simulink model "dspblr7_Ave"  (R2018a)
settings: Solver=VariableStepAuto  StartTime=0.0  StopTime=100e-6  RelTol=1e-3
libraries: xbsIndex_r4 x61, xrbsSSR_Library x17, dspsigattribs x1, hdlsllib x1, simulink x1
(part 2 of 2)

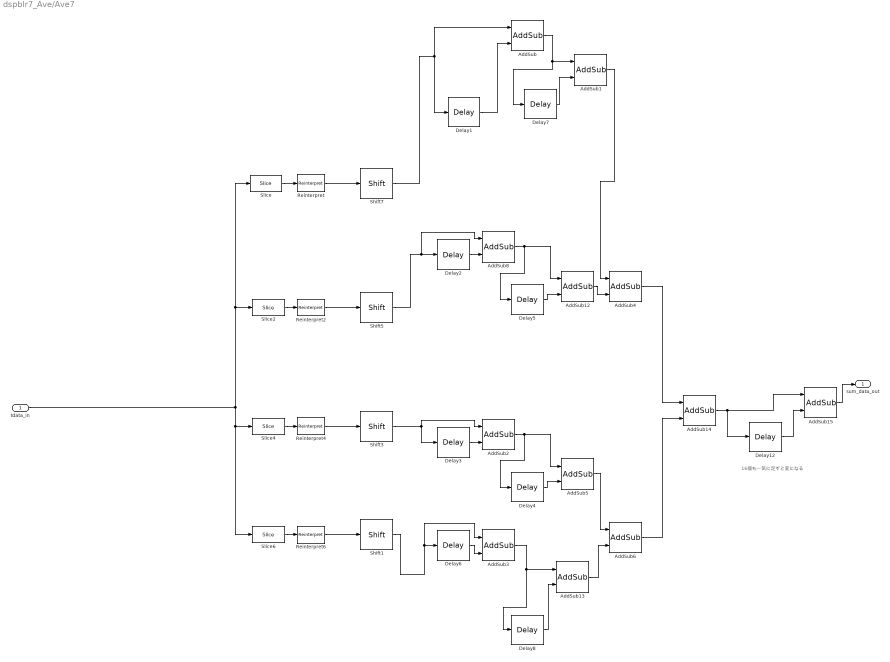
== system dspblr7_Ave/Ave7 ==
  note: 16個も一気に足すと変になる
  tdata_in : Inport
  AddSub{,1..3,8,12..15} (9 alike) : xbsIndex_r4/AddSub  mode=Addition  use_carryin=off  use_carryout=off  en=off  latency=0  precision=User Defined  arith_type="Signed  (2's comp)"  n_bits=17  bin_pt=4  quantization=Truncate  overflow=Wrap  use_behavioral_HDL=off  hw_selection=Fabric  pipelined=off  dbl_ovrd=off  block_type=addsub
  AddSub4 : xbsIndex_r4/AddSub  mode=Addition  use_carryin=off  use_carryout=off  en=off  latency=0  precision=Full  arith_type="Signed  (2's comp)"  n_bits=18  bin_pt=4  quantization=Truncate  overflow=Wrap  use_behavioral_HDL=off  hw_selection=Fabric  pipelined=off  dbl_ovrd=off  block_type=addsub
  AddSub5 : xbsIndex_r4/AddSub  mode=Addition  use_carryin=off  use_carryout=off  en=off  latency=0  precision=Full  arith_type="Signed  (2's comp)"  n_bits=18  bin_pt=4  quantization=Truncate  overflow=Wrap  use_behavioral_HDL=off  hw_selection=Fabric  pipelined=off  dbl_ovrd=off  block_type=addsub
  AddSub6 : xbsIndex_r4/AddSub  mode=Addition  use_carryin=off  use_carryout=off  en=off  latency=0  precision=User Defined  arith_type="Signed  (2's comp)"  n_bits=19  bin_pt=4  quantization=Truncate  overflow=Wrap  use_behavioral_HDL=off  hw_selection=Fabric  pipelined=off  dbl_ovrd=off  block_type=addsub
  Delay{1..3,6} (4 alike) : xbsIndex_r4/Delay  rst=off  infoeditControl=Selection of Reset will increase slice count due to use of real FFs and instead of SRLs  en=off  latency=1  reg_retiming=off  dbl_ovrd=off  block_type=delay
  Delay12 : xbsIndex_r4/Delay  rst=off  infoeditControl=Selection of Reset will increase slice count due to use of real FFs and instead of SRLs  en=off  latency=4  reg_retiming=off  dbl_ovrd=off  block_type=delay
  Delay{4..5,7..8} (4 alike) : xbsIndex_r4/Delay  rst=off  infoeditControl=Selection of Reset will increase slice count due to use of real FFs and instead of SRLs  en=off  latency=2  reg_retiming=off  dbl_ovrd=off  block_type=delay
  Reinterpret{,2,4,6} (4 alike) : xbsIndex_r4/Reinterpret  force_arith_type=on  arith_type="Signed  (2's comp)"  force_bin_pt=on  bin_pt=4  block_type=reinterpret
  Shift{1,3,5,7} (4 alike) : xbsIndex_r4/Shift  shift_dir=Right  shift_bits=5  en=off  latency=1  precision=Full  arith_type="Signed  (2's comp)"  n_bits=16  bin_pt=14  quantization=Truncate  overflow=Wrap  dbl_ovrd=off  block_type=shift
  Slice : xbsIndex_r4/Slice  nbits=16  boolean_output=off  mode=Two Bit Locations  bit1=15  base1=LSB of Input  bit0=0  base0=LSB of Input  dbl_ovrd=off  block_type=slice
  Slice2 : xbsIndex_r4/Slice  nbits=16  boolean_output=off  mode=Two Bit Locations  bit1=47  base1=LSB of Input  bit0=32  base0=LSB of Input  dbl_ovrd=off  block_type=slice
  Slice4 : xbsIndex_r4/Slice  nbits=16  boolean_output=off  mode=Two Bit Locations  bit1=79  base1=LSB of Input  bit0=64  base0=LSB of Input  dbl_ovrd=off  block_type=slice
  Slice6 : xbsIndex_r4/Slice  nbits=16  boolean_output=off  mode=Two Bit Locations  bit1=111  base1=LSB of Input  bit0=96  base0=LSB of Input  dbl_ovrd=off  block_type=slice
  sum_data_out : Outport  OutDataTypeStr=fixdt(1,19,4)
  wires:
  Slice4/1 -> Reinterpret4/1
  Reinterpret6/1 -> Shift1/1
  AddSub14/1 -> Delay12/1, AddSub15/1
  AddSub13/1 -> AddSub6/2
  AddSub4/1 -> AddSub14/1
  AddSub8/1 -> Delay5/1, AddSub12/1
  Reinterpret4/1 -> Shift3/1
  Delay7/1 -> AddSub1/2
  AddSub6/1 -> AddSub14/2
  Slice2/1 -> Reinterpret2/1
  Slice/1 -> Reinterpret/1
  AddSub5/1 -> AddSub6/1
  Slice6/1 -> Reinterpret6/1
  Shift5/1 -> AddSub8/1, Delay2/1
  Delay2/1 -> AddSub8/2
  tdata_in/1 -> Slice/1, Slice2/1, Slice4/1, Slice6/1
  AddSub1/1 -> AddSub4/1
  Shift7/1 -> AddSub/1, Delay1/1
  Delay1/1 -> AddSub/2
  AddSub/1 -> Delay7/1, AddSub1/1
  Reinterpret2/1 -> Shift5/1
  Delay5/1 -> AddSub12/2
  Reinterpret/1 -> Shift7/1
  AddSub12/1 -> AddSub4/2
  AddSub15/1 -> sum_data_out/1
  Delay12/1 -> AddSub15/2
  AddSub2/1 -> AddSub5/1, Delay4/1
  Delay3/1 -> AddSub2/2
  Shift3/1 -> Delay3/1, AddSub2/1
  Delay4/1 -> AddSub5/2
  AddSub3/1 -> Delay8/1, AddSub13/1
  Delay6/1 -> AddSub3/2
  Shift1/1 -> AddSub3/1, Delay6/1
  Delay8/1 -> AddSub13/2

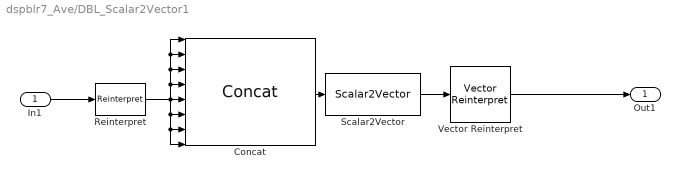
== system dspblr7_Ave/DBL_Scalar2Vector1 ==
  In1 : Inport
  Concat : xbsIndex_r4/Concat  num_inputs=8  dbl_ovrd=off  block_type=concat
  Reinterpret : xbsIndex_r4/Reinterpret  force_arith_type=on  arith_type=Unsigned  force_bin_pt=on  bin_pt=0  block_type=reinterpret
  Scalar2Vector : xrbsSSR_Library/Scalar2Vector  Width=16  sg_ssr=8  sg_ssr_prev=8  sg_ssr_name=vect_Scalar2Vector  block_type=scalar2vector_ssr
      settings: SourceProductName=Xilinx SSR Blockset
  Vector Reinterpret : xrbsSSR_Library/Vector Reinterpret  sg_ssr=8  sg_ssr_prev=8  force_arith_type=on  arith_type="Signed  (2's comp)"  force_bin_pt=on  bin_pt=4  block_type=reinterpret_ssr
      settings: SourceProductName=Xilinx SSR Blockset  infoedit="The Vector Reinterpret block Changes vector input signal type without altering the binary representation. You can change the signal between signed and unsigned, and relocate the binary point.<br><br>Hardware notes: In hardware this block costs nothing.<br><br>Example:  Suppose the input is 6 bits wide, signed, with 2 fractional bits, and the output is forced to unsigned with 0 fractional bits.  Then an input of -2.0 (1110.00 in binary 2's complement) becomes an output of 56 (111000 in binary)."
  Out1 : Outport
  wires:
  In1/1 -> Reinterpret/1
  Vector Reinterpret/1 -> Out1/1
  Reinterpret/1 -> Concat/1, Concat/2, Concat/3, Concat/4, Concat/8, Concat/7, Concat/6, Concat/5
  Concat/1 -> Scalar2Vector/1
  Scalar2Vector/1 -> Vector Reinterpret/1

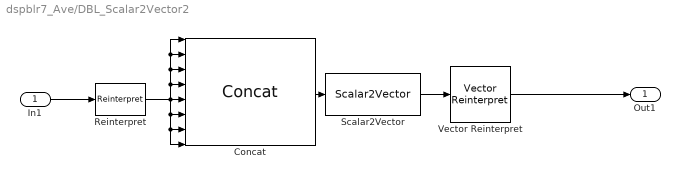
== system dspblr7_Ave/DBL_Scalar2Vector2 ==
  In1 : Inport
  Concat : xbsIndex_r4/Concat  num_inputs=8  dbl_ovrd=off  block_type=concat
  Reinterpret : xbsIndex_r4/Reinterpret  force_arith_type=on  arith_type=Unsigned  force_bin_pt=on  bin_pt=0  block_type=reinterpret
  Scalar2Vector : xrbsSSR_Library/Scalar2Vector  Width=16  sg_ssr=8  sg_ssr_prev=8  sg_ssr_name=vect_Scalar2Vector  block_type=scalar2vector_ssr
      settings: SourceProductName=Xilinx SSR Blockset
  Vector Reinterpret : xrbsSSR_Library/Vector Reinterpret  sg_ssr=8  sg_ssr_prev=8  force_arith_type=on  arith_type="Signed  (2's comp)"  force_bin_pt=on  bin_pt=4  block_type=reinterpret_ssr
      settings: SourceProductName=Xilinx SSR Blockset  infoedit="The Vector Reinterpret block Changes vector input signal type without altering the binary representation. You can change the signal between signed and unsigned, and relocate the binary point.<br><br>Hardware notes: In hardware this block costs nothing.<br><br>Example:  Suppose the input is 6 bits wide, signed, with 2 fractional bits, and the output is forced to unsigned with 0 fractional bits.  Then an input of -2.0 (1110.00 in binary 2's complement) becomes an output of 56 (111000 in binary)."
  Out1 : Outport
  wires:
  In1/1 -> Reinterpret/1
  Vector Reinterpret/1 -> Out1/1
  Reinterpret/1 -> Concat/1, Concat/2, Concat/3, Concat/4, Concat/8, Concat/7, Concat/6, Concat/5
  Concat/1 -> Scalar2Vector/1
  Scalar2Vector/1 -> Vector Reinterpret/1

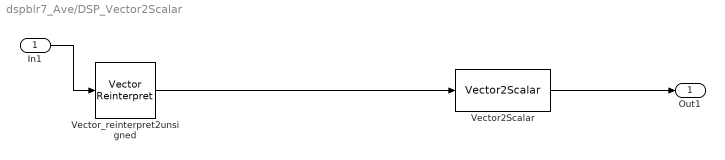
== system dspblr7_Ave/DSP_Vector2Scalar ==
  In1 : Inport
  Vector2Scalar : xrbsSSR_Library/Vector2Scalar  sg_ssr=8  sg_ssr_prev=8  sg_ssr_name=vect_Vector2Scalar  block_type=vector2scalar_ssr
      settings: SourceProductName=Xilinx SSR Blockset
  Vector_reinterpret2unsigned : xrbsSSR_Library/Vector Reinterpret  sg_ssr=8  sg_ssr_prev=8  force_arith_type=on  arith_type=Unsigned  force_bin_pt=on  bin_pt=0  block_type=reinterpret_ssr
      settings: SourceProductName=Xilinx SSR Blockset  infoedit="The Vector Reinterpret block Changes vector input signal type without altering the binary representation. You can change the signal between signed and unsigned, and relocate the binary point.<br><br>Hardware notes: In hardware this block costs nothing.<br><br>Example:  Suppose the input is 6 bits wide, signed, with 2 fractional bits, and the output is forced to unsigned with 0 fractional bits.  Then an input of -2.0 (1110.00 in binary 2's complement) becomes an output of 56 (111000 in binary)."
  Out1 : Outport
  wires:
  In1/1 -> Vector_reinterpret2unsigned/1
  Vector_reinterpret2unsigned/1 -> Vector2Scalar/1
  Vector2Scalar/1 -> Out1/1

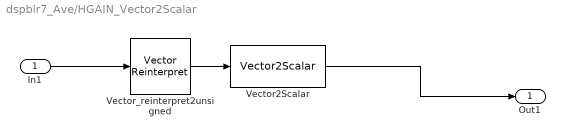
== system dspblr7_Ave/HGAIN_Vector2Scalar ==
  In1 : Inport
  Vector2Scalar : xrbsSSR_Library/Vector2Scalar  sg_ssr=8  sg_ssr_prev=8  sg_ssr_name=vect_Vector2Scalar  block_type=vector2scalar_ssr
      settings: SourceProductName=Xilinx SSR Blockset
  Vector_reinterpret2unsigned : xrbsSSR_Library/Vector Reinterpret  sg_ssr=8  sg_ssr_prev=8  force_arith_type=on  arith_type=Unsigned  force_bin_pt=on  bin_pt=0  block_type=reinterpret_ssr
      settings: SourceProductName=Xilinx SSR Blockset  infoedit="The Vector Reinterpret block Changes vector input signal type without altering the binary representation. You can change the signal between signed and unsigned, and relocate the binary point.<br><br>Hardware notes: In hardware this block costs nothing.<br><br>Example:  Suppose the input is 6 bits wide, signed, with 2 fractional bits, and the output is forced to unsigned with 0 fractional bits.  Then an input of -2.0 (1110.00 in binary 2's complement) becomes an output of 56 (111000 in binary)."
  Out1 : Outport
  wires:
  Vector_reinterpret2unsigned/1 -> Vector2Scalar/1
  In1/1 -> Vector_reinterpret2unsigned/1
  Vector2Scalar/1 -> Out1/1

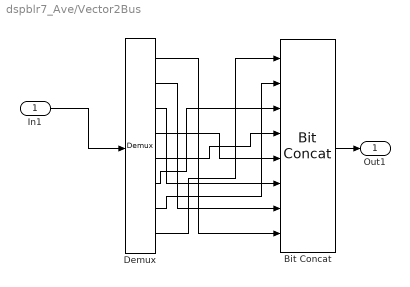
== system dspblr7_Ave/Vector2Bus ==
  In1 : Inport
  Bit Concat : hdlsllib/Logic and Bit Operations/Bit Concat  numInputs=8
      settings: SourceProductName=HDL Coder  SourceProductBaseCode=HD
  Demux : Demux  Outputs=8
  Out1 : Outport
  wires:
  Demux/1 -> Bit Concat/8
  Demux/8 -> Bit Concat/1
  Demux/3 -> Bit Concat/6
  Bit Concat/1 -> Out1/1
  Demux/7 -> Bit Concat/2
  Demux/4 -> Bit Concat/5
  Demux/2 -> Bit Concat/7
  Demux/6 -> Bit Concat/3
  Demux/5 -> Bit Concat/4
  In1/1 -> Demux/1
